simulink model "LQG_KF_P2andW_sim"  (Simulink 7.5)
settings: Solver=ode15s  StartTime=0.0  StopTime=10000  RelTol=1e-8
undefined symbols (not defined in the file or in its folder): Du, K, kest, u0, y0
settings Model: Creator=jahansha  LastModifiedBy=tereseva

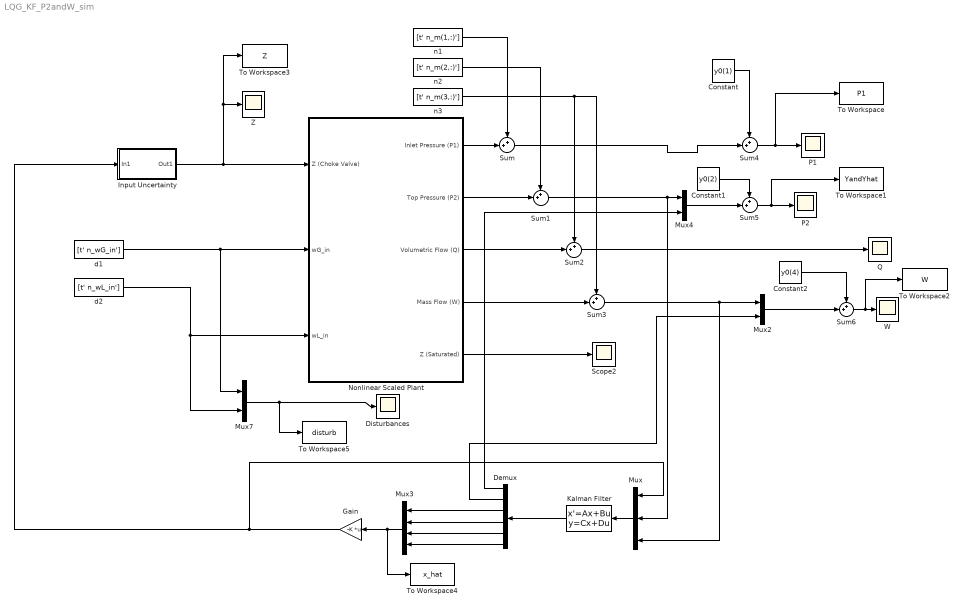
== system LQG_KF_P2andW_sim ==
  Constant : Constant  Value=y0(1)
  Constant1 : Constant  Value=y0(2)
  Constant2 : Constant  Value=y0(4)
  Demux : Demux  Outputs=6
  Disturbances : Scope
      settings: TimeRange=8000  YMin=1.38778e-017  YMax=0.275  SaveName=ScopeData5
  Gain : Gain  Gain=-K  Multiplication=Matrix(K*u)
  Input Uncertainty : Subsystem
  Kalman Filter : StateSpace  A=kest.a  B=kest.b  C=kest.c  D=kest.d
  Mux : Mux  Inputs=3
  Mux2 : Mux  Inputs=2
  Mux3 : Mux
  Mux4 : Mux  Inputs=2
  Mux7 : Mux  Inputs=2
  Nonlinear Scaled Plant : Subsystem
  P1 : Scope
      settings: YMin=-0.1  YMax=0.06
  P2 : Scope
      settings: TimeRange=1000  YMin=0.02  YMax=0.23  SaveName=ScopeData3
  Q : Scope
      settings: TimeRange=10000  YMin=-2.5  YMax=4  SaveName=ScopeData4
  Scope2 : Scope
      settings: TimeRange=8000  YMin=0.105  YMax=0.113  SaveName=ScopeData7
  Sum{,1..6} (7 alike) : Sum  Inputs=++|
  To Workspace : ToWorkspace  VariableName=P1  SampleTime=-1  SaveFormat=Array
  To Workspace1 : ToWorkspace  VariableName=YandYhat  SampleTime=-1  SaveFormat=Array
  To Workspace2 : ToWorkspace  VariableName=W  SampleTime=-1  SaveFormat=Array
  To Workspace3 : ToWorkspace  VariableName=Z  SampleTime=-1  SaveFormat=Array
  To Workspace4 : ToWorkspace  VariableName=x_hat  SampleTime=-1  SaveFormat=Structure
  To Workspace5 : ToWorkspace  VariableName=disturb  SampleTime=-1  SaveFormat=Array
  W : Scope
      settings: YMin=0.225  YMax=0.55  SaveName=ScopeData2
  Z : Scope
      settings: TimeRange=1000  YMin=-0.0092  YMax=-0.0076
  d1 : FromWorkspace  VariableName=[t' n_wG_in']  SampleTime=0
  d2 : FromWorkspace  VariableName=[t' n_wL_in']  SampleTime=0
  n1 : FromWorkspace  VariableName=[t' n_m(1,:)']  SampleTime=0
  n2 : FromWorkspace  VariableName=[t' n_m(2,:)']  SampleTime=0
  n3 : FromWorkspace  VariableName=[t' n_m(3,:)']  SampleTime=0
  wires:
  Nonlinear Scaled Plant/2(Top Pressure (P2)) -> Sum1/2
  Nonlinear Scaled Plant/3(Volumetric Flow (Q)) -> Sum2/2
  Nonlinear Scaled Plant/1(Inlet Pressure (P1)) -> Sum/2
  Input Uncertainty/1(Out1) -> Nonlinear Scaled Plant/1(Z (Choke Valve)), Z/1, To Workspace3/1
  Mux7/1 -> Disturbances/1, To Workspace5/1
  d1/1 -> Mux7/1, Nonlinear Scaled Plant/2(wG_in)
  d2/1 -> Mux7/2, Nonlinear Scaled Plant/3(wL_in)
  Nonlinear Scaled Plant/4(Mass Flow (W)) -> Sum3/2
  Nonlinear Scaled Plant/5(Z (Saturated)) -> Scope2/1
  Mux/1 -> Kalman Filter/1
  Kalman Filter/1 -> Demux/1
  Demux/2 -> Mux2/2
  Sum2/1 -> Q/1
  Demux/3 -> Mux3/1
  Demux/4 -> Mux3/2
  Demux/5 -> Mux3/3
  Demux/6 -> Mux3/4
  Mux3/1 -> Gain/1, To Workspace4/1
  Gain/1 -> Input Uncertainty/1(In1), Mux/1
  n1/1 -> Sum/1
  n2/1 -> Sum1/1
  n3/1 -> Sum2/1, Sum3/1
  Sum3/1 -> Mux2/1, Mux/3
  Sum4/1 -> P1/1, To Workspace/1
  Constant/1 -> Sum4/1
  Constant1/1 -> Sum5/1
  Sum5/1 -> P2/1, To Workspace1/1
  Mux2/1 -> Sum6/2
  Sum6/1 -> W/1, To Workspace2/1
  Constant2/1 -> Sum6/1
  Mux4/1 -> Sum5/2
  Sum1/1 -> Mux4/1, Mux/2
  Demux/1 -> Mux4/2
  Sum/1 -> Sum4/2

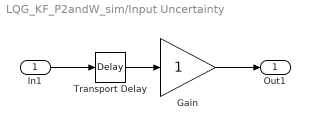
== system LQG_KF_P2andW_sim/Input Uncertainty ==
  In1 : Inport
  Gain : Gain
  Transport Delay : TransportDelay  DelayTime=0
  Out1 : Outport
  wires:
  Transport Delay/1 -> Gain/1
  In1/1 -> Transport Delay/1
  Gain/1 -> Out1/1

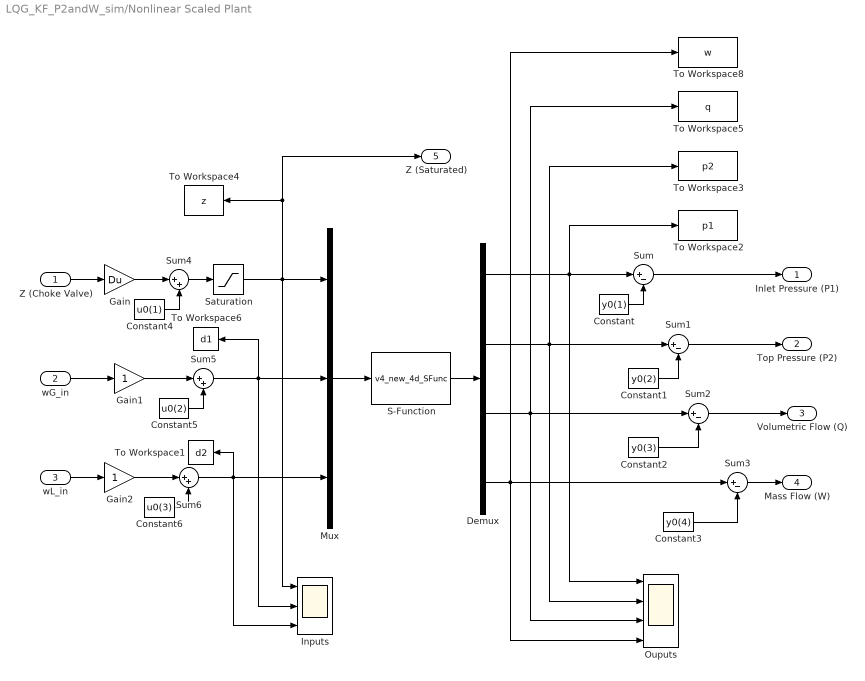
== system LQG_KF_P2andW_sim/Nonlinear Scaled Plant ==
  Z (Choke Valve) : Inport
  wG_in : Inport  Port=2
  wL_in : Inport  Port=3
  Constant : Constant  Value=y0(1)
  Constant1 : Constant  Value=y0(2)
  Constant2 : Constant  Value=y0(3)
  Constant3 : Constant  Value=y0(4)
  Constant4 : Constant  Value=u0(1)
  Constant5 : Constant  Value=u0(2)
  Constant6 : Constant  Value=u0(3)
  Demux : Demux
  Gain : Gain  Gain=Du
  Gain1 : Gain
  Gain2 : Gain
  Inputs : Scope  NumInputPorts=3
      settings: TimeRange=8000  YMin=-1~-5~-5  YMax=1~5~5  SaveName=ScopeData9
  Mux : Mux  Inputs=3
  Ouputs : Scope  NumInputPorts=4
      settings: TimeRange=8000  YMin=-1~-5~-5~-5  YMax=1~5~5~5  SaveName=ScopeData10
  S-Function : S-Function  FunctionName=v4_new_4d_SFunc  EnableBusSupport=off
  Saturation : Saturate  UpperLimit=1  LowerLimit=0
  Sum{,1..3} (4 alike) : Sum  Inputs=|+-
  Sum4 : Sum  Inputs=|++
  Sum5 : Sum  Inputs=|++
  Sum6 : Sum  Inputs=|++
  To Workspace1 : ToWorkspace  VariableName=d2  SampleTime=-1  SaveFormat=Array
  To Workspace2 : ToWorkspace  VariableName=p1  SampleTime=-1  SaveFormat=Array
  To Workspace3 : ToWorkspace  VariableName=p2  SampleTime=-1  SaveFormat=Array
  To Workspace4 : ToWorkspace  VariableName=z  SampleTime=-1  SaveFormat=Array
  To Workspace5 : ToWorkspace  VariableName=q  SampleTime=-1  SaveFormat=Array
  To Workspace6 : ToWorkspace  VariableName=d1  SampleTime=-1  SaveFormat=Array
  To Workspace8 : ToWorkspace  VariableName=w  SampleTime=-1  SaveFormat=Array
  Inlet Pressure (P1) : Outport
  Top Pressure (P2) : Outport  Port=2
  Volumetric Flow (Q) : Outport  Port=3
  Mass Flow (W) : Outport  Port=4
  Z (Saturated) : Outport  Port=5
  wires:
  Mux/1 -> S-Function/1
  S-Function/1 -> Demux/1
  Demux/1 -> Ouputs/1, Sum/1, To Workspace2/1
  Constant/1 -> Sum/2
  Demux/2 -> Sum1/1, Ouputs/2, To Workspace3/1
  Constant1/1 -> Sum1/2
  Demux/3 -> Sum2/1, Ouputs/3, To Workspace5/1
  Constant2/1 -> Sum2/2
  Constant3/1 -> Sum3/2
  Sum/1 -> Inlet Pressure (P1)/1
  Sum1/1 -> Top Pressure (P2)/1
  Sum2/1 -> Volumetric Flow (Q)/1
  Demux/4 -> Sum3/1, Ouputs/4, To Workspace8/1
  Sum3/1 -> Mass Flow (W)/1
  Constant4/1 -> Sum4/2
  Z (Choke Valve)/1 -> Gain/1
  Gain/1 -> Sum4/1
  Constant5/1 -> Sum5/2
  Gain1/1 -> Sum5/1
  wG_in/1 -> Gain1/1
  Sum5/1 -> Mux/2, Inputs/2, To Workspace6/1
  Constant6/1 -> Sum6/2
  Gain2/1 -> Sum6/1
  wL_in/1 -> Gain2/1
  Sum6/1 -> Mux/3, Inputs/3, To Workspace1/1
  Saturation/1 -> Mux/1, Inputs/1, Z (Saturated)/1, To Workspace4/1
  Sum4/1 -> Saturation/1
